simulink model "PID_basic_block_Controller"  (R2020a)
settings: Solver=ode45  StartTime=0.0  StopTime=120  RelTol=1e-3
settings Model: DataDictionary=init_values.sldd  Creator=Prateek  LastModifiedBy=Prateek
settings DataIOCC: SaveOutput=off  SaveTime=off

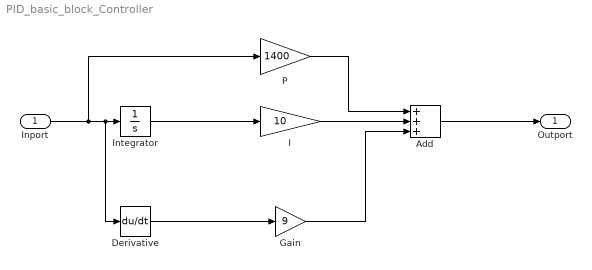
== system PID_basic_block_Controller ==
  Inport : Inport  OutDataTypeStr=double  PortDimensions=1  SampleTime=0
  Add : Sum  Inputs=+++
  Derivative : Derivative
  Gain : Gain  Gain=9
  I : Gain  Gain=10
  Integrator : Integrator
  P : Gain  Gain=1400
  Outport : Outport  OutDataTypeStr=double  PortDimensions=1  SampleTime=0
  wires:
  Inport/1 -> Integrator/1, Derivative/1, P/1
  P/1 -> Add/1
  I/1 -> Add/2
  Add/1 -> Outport/1
  Integrator/1 -> I/1
  Derivative/1 -> Gain/1
  Gain/1 -> Add/3
